simulink model "Halfcarmodelwithvaryingroadprofiles"  (R2022b)
settings: Solver=VariableStepAuto  StartTime=0.0  StopTime=10.0  RelTol=1e-3
undefined symbols (not defined in the file): a1, a2, c1, c2, Iy, k1, k2, k_t1, k_t2, m, m1, m2
settings Model: Creator=abhilashbharadwaj  LastModifiedBy=abhilashbharadwaj

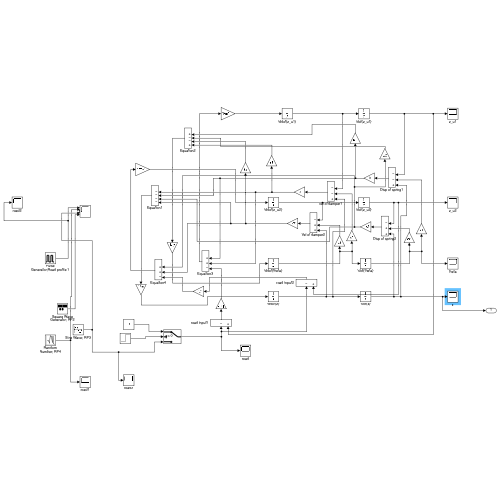
[thumbnail: Simulink's stored preview of the top-level diagram]
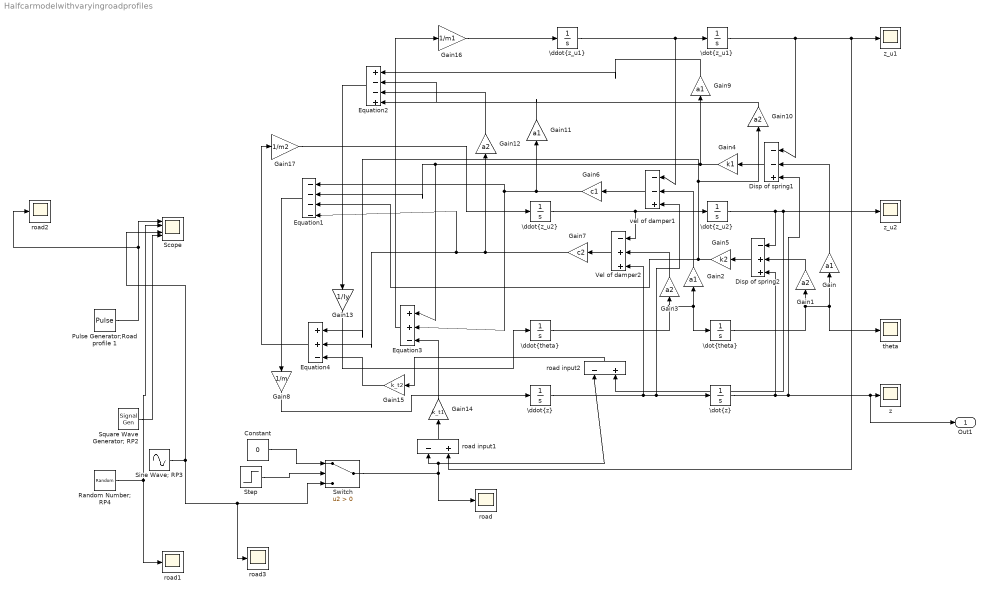
== system Halfcarmodelwithvaryingroadprofiles ==
  Constant : Constant  Value=0
  Disp of spring1 : Sum  Inputs=|--+
  Disp of spring2 : Sum  Inputs=|-++
  Equation1 : Sum  Inputs=|----
  Equation2 : Sum  Inputs=|+--+
  Equation3 : Sum  Inputs=|++-
  Equation4 : Sum  Inputs=|++-
  Gain{,2,9,11} (4 alike) : Gain  Gain=a1
  Gain{1,3,10,12} (4 alike) : Gain  Gain=a2
  Gain13 : Gain  Gain=1/Iy
  Gain14 : Gain  Gain=k_t1
  Gain15 : Gain  Gain=k_t2
  Gain16 : Gain  Gain=1/m1
  Gain17 : Gain  Gain=1/m2
  Gain4 : Gain  Gain=k1
  Gain5 : Gain  Gain=k2
  Gain6 : Gain  Gain=c1
  Gain7 : Gain  Gain=c2
  Gain8 : Gain  Gain=1/m
  Pulse Generator;Road profile 1 : DiscretePulseGenerator  PulseType=Time based  Amplitude=0.25  PulseWidth=15  PhaseDelay=1
  Random Number; RP4 : RandomNumber  Variance=0.25  SampleTime=0.8
  Scope : Scope  NumInputPorts=5
  Sine Wave; RP3 : Sin  Amplitude=0.28  Frequency=0.628  SampleTime=0
  Square Wave Generator; RP2 : SignalGenerator  WaveForm=sawtooth  Amplitude=0.28  Units=rad/sec
  Step : Step  Time=3.2  After=10  SampleTime=0
  Switch : Switch  Criteria=u2 > Threshold  SaturateOnIntegerOverflow=off  InputSameDT=off
  Vel of damper2 : Sum  Inputs=|-++
  "\\ddot{theta}" : Integrator
  "\\ddot{z_u1}" : Integrator
  "\\ddot{z_u2}" : Integrator
  "\\ddot{z}" : Integrator
  "\\dot{theta}" : Integrator
  "\\dot{z_u1}" : Integrator
  "\\dot{z_u2}" : Integrator
  "\\dot{z}" : Integrator
  road{,1..3} (4 alike) : Scope
  road input1 : Sum  Inputs=|-+
  road input2 : Sum  Inputs=|-+
  theta : Scope
  vel of damper1 : Sum  Inputs=|--+
  z : Scope
  z_u1 : Scope
  z_u2 : Scope
  Out1 : Outport
  wires:
  "\\ddot{z_u2}"/1 -> Vel of damper2/1, "\\dot{z_u2}"/1
  "\\ddot{theta}"/1 -> Gain3/1, Gain2/1, "\\dot{theta}"/1
  "\\ddot{z}"/1 -> vel of damper1/3, "\\dot{z}"/1, Vel of damper2/3
  "\\dot{z_u1}"/1 -> road input1/2, z_u1/1, Disp of spring1/1
  "\\dot{z_u2}"/1 -> road input2/2, z_u2/1, Disp of spring2/1
  "\\dot{theta}"/1 -> Gain1/1, Gain/1, theta/1
  "\\dot{z}"/1 -> Disp of spring1/3, Out1/1, z/1, Disp of spring2/3
  Gain/1 -> Disp of spring1/2
  Gain1/1 -> Disp of spring2/2
  Gain2/1 -> vel of damper1/2
  Gain3/1 -> Vel of damper2/2
  Disp of spring1/1 -> Gain4/1
  Disp of spring2/1 -> Gain5/1
  vel of damper1/1 -> Gain6/1
  Vel of damper2/1 -> Gain7/1
  Gain6/1 -> Equation1/1, Equation3/2, Gain11/1
  Gain7/1 -> Equation1/4, Equation4/2, Gain12/1
  Gain5/1 -> Gain10/1, Equation4/1, Equation1/3
  Equation1/1 -> Gain8/1
  "\\ddot{z_u1}"/1 -> "\\dot{z_u1}"/1, vel of damper1/1
  Gain4/1 -> Equation1/2, Equation3/1, Gain9/1
  Gain11/1 -> Equation2/4
  Gain9/1 -> Equation2/1
  Gain12/1 -> Equation2/3
  Gain10/1 -> Equation2/2
  Equation2/1 -> Gain13/1
  Gain13/1 -> "\\ddot{theta}"/1
  road input1/1 -> Gain14/1
  Gain14/1 -> Equation3/3
  Gain8/1 -> "\\ddot{z}"/1
  Equation3/1 -> Gain16/1
  road input2/1 -> Gain15/1
  Gain15/1 -> Equation4/3
  Gain16/1 -> "\\ddot{z_u1}"/1
  Equation4/1 -> Gain17/1
  Gain17/1 -> "\\ddot{z_u2}"/1
  Step/1 -> Switch/2
  Sine Wave; RP3/1 -> road3/1, Switch/3, Scope/4
  Constant/1 -> Switch/1
  Switch/1 -> road/1, road input2/1, road input1/1
  Square Wave Generator; RP2/1 -> Scope/5
  Pulse Generator;Road profile 1/1 -> Scope/1, road2/1
  Random Number; RP4/1 -> road1/1, Scope/2
